simulink library "SunPosition"  (R2014b)
settings: Solver=ode45  StartTime=0.0  StopTime=10.0  RelTol=1e-3
undefined symbols (not defined in the file): ConfParam
libraries: SunDirection x1
settings Model: Creator=Hp  LastModifiedBy=Hp

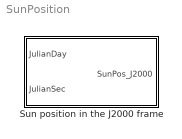
== system SunPosition ==
  Sun position in the J2000 frame : Subsystem

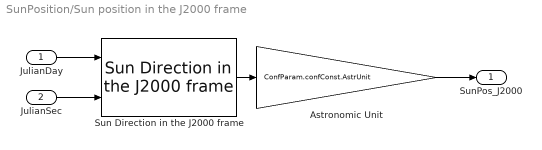
== system SunPosition/Sun position in the J2000 frame ==
  JulianDay : Inport
  JulianSec : Inport  Port=2
  Astronomic Unit : Gain  Gain=ConfParam.confConst.AstrUnit
  Sun Direction in the J2000 frame : SunDirection/Sun Direction in the J2000 frame
  SunPos_J2000 : Outport
  wires:
  Sun Direction in the J2000 frame/1 -> Astronomic Unit/1
  JulianSec/1 -> Sun Direction in the J2000 frame/2
  JulianDay/1 -> Sun Direction in the J2000 frame/1
  Astronomic Unit/1 -> SunPos_J2000/1
